simulink subsystem "Week2CarKinematics"  (R2024b)
settings: Solver=VariableStepAuto  StartTime=0.0  StopTime=10.0  RelTol=1e-3
undefined symbols (not defined in the file or in its folder): vehicleData
settings Model: Creator=btagl  LastModifiedBy=btagl

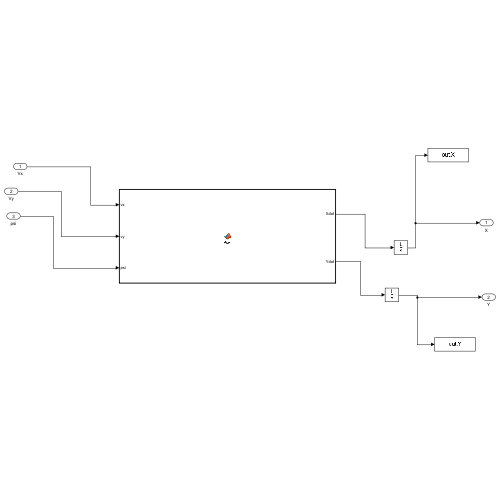
[thumbnail: Simulink's stored preview of the top-level diagram]
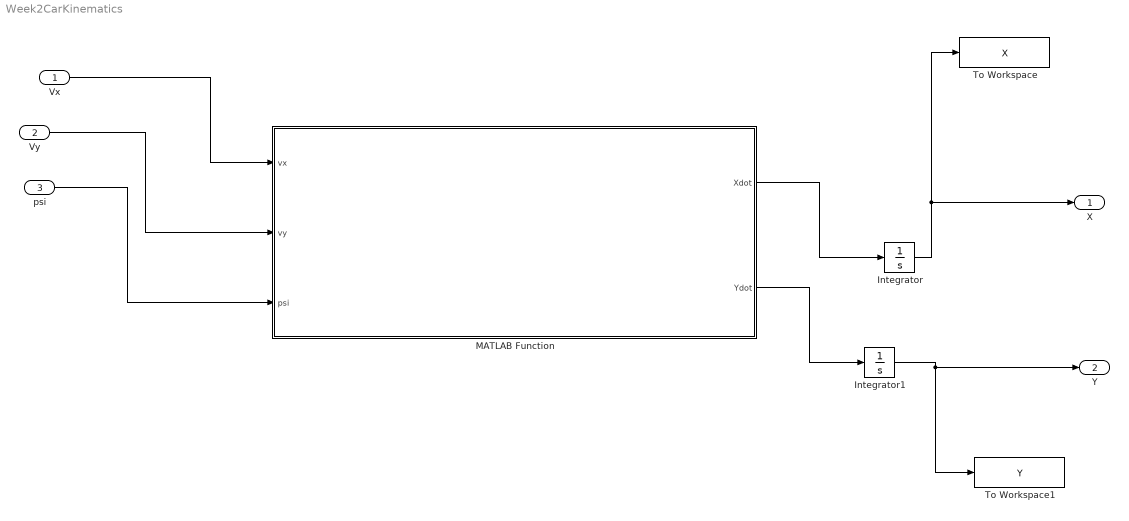
== system Week2CarKinematics ==
  Vx : Inport
  Vy : Inport  Port=2
  psi : Inport  Port=3
  Integrator : Integrator  InitialCondition=vehicleData.init.X0
  Integrator1 : Integrator  InitialCondition=vehicleData.init.Y0
  MATLAB Function : MATLAB Function  TreatAsAtomicUnit=on
  To Workspace : ToWorkspace  VariableName=X  SaveFormat=Timeseries  SampleTime=-1
  To Workspace1 : ToWorkspace  VariableName=Y  SaveFormat=Timeseries  SampleTime=-1
  X : Outport
  Y : Outport  Port=2
  wires:
  Vy/1 -> MATLAB Function/2(vy)
  psi/1 -> MATLAB Function/3(psi)
  Vx/1 -> MATLAB Function/1(vx)
  Integrator/1 -> To Workspace/1, X/1
  Integrator1/1 -> Y/1, To Workspace1/1
  MATLAB Function/1(Xdot) -> Integrator/1
  MATLAB Function/2(Ydot) -> Integrator1/1

== matlab function Week2CarKinematics/MATLAB Function ==
  data: Xdot output; Ydot output; vx input; vy input; psi input
function [Xdot, Ydot] = fcn(vx, vy, psi)
    temp = TF(psi) * [vx;vy]; 
    Xdot = temp(1);
    Ydot = temp(2);
end

function y = TF(psi)
    y = [cos(psi), -sin(psi); sin(psi), cos(psi)];
end
